simulink library "RefChMixer"  (R2022b)
settings: Solver=VariableStepAuto  StartTime=0.0  StopTime=10.0  RelTol=1e-3
undefined symbols (not defined in the file or in its folder): mixing_gains_fader, mixing_gains_normal, tune_fade_pos
libraries: RefChMixerBtc x1
settings Model: Creator=nikunj.tapodhan  LastModifiedBy=kl13806
settings SolverCC: AlgebraicLoopSolver=TrustRegion
settings DebuggingCC: UnconnectedInputMsg=warning  UnconnectedOutputMsg=warning  UnconnectedLineMsg=warning  SFMachineParentedDataDiag=warning  ArithmeticOperatorsInVariantConditions=warning
settings ModelReferenceCC: EnableRefExpFcnMdlSchedulingChecks=on
settings SFSimCC: CustomCodeUndefinedFunction=UseInterfaceOnly
settings RTWCC: DLArmComputeVersion=19.05

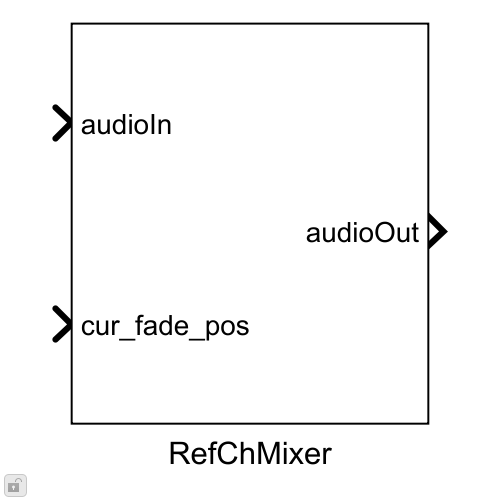
[thumbnail: Simulink's stored preview of the top-level diagram]
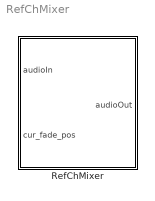
== system RefChMixer ==
  RefChMixer : Subsystem  mask{includeFade=on, mixingGainsNormal=mixing_gains_normal, mixingGainsFader=mixing_gains_fader, tuneFadePos=tune_fade_pos}
      mask prompts: includeFade "Include Fader flag"; mixingGainsNormal "Mixing gain matrix - normal"; mixingGainsFader "Mixing gain matrix - fader"; tuneFadePos "Tune Fader position"
      mask help: Iclude fader flag is to select whether fader function is to be added or not for generating reference output
      mask init:
      | blkh = gcbh;
      | % Copy discrete mask parameters into a classdef object
      | InnerLinkConfig = RefChMixerConfig;
      | InnerLinkConfig.IncludeFade = includeFade;
      | InnerLinkConfig.DefaultMixingGainsNormal = mixingGainsNormal;
      | InnerLinkConfig.DefaultMixingGainsFader = mixingGainsFader;
      | InnerLinkConfig.DefaultTuneFadePos = tuneFadePos;

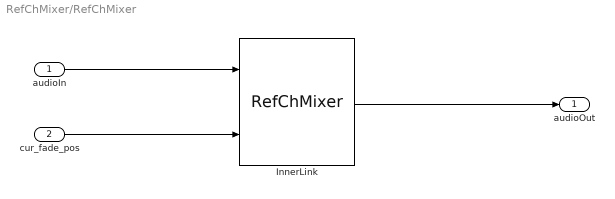
== system RefChMixer/RefChMixer ==
  audioIn : Inport
  cur_fade_pos : Inport  Port=2
  InnerLink : RefChMixerBtc/RefChMixer  Config=InnerLinkConfig  FeatureName=refChMixer
      settings: SourceProductName=Bose Blocklib
  audioOut : Outport
  wires:
  InnerLink/1 -> audioOut/1
  audioIn/1 -> InnerLink/1
  cur_fade_pos/1 -> InnerLink/2
